simulink model "feedback_control_basic"  (R2017a)
settings: Solver=VariableStepAuto  StartTime=0.0  StopTime=10.0  RelTol=1e-3
libraries: cstblocks x5
settings Model: Creator=Roman  LastModifiedBy=Roman

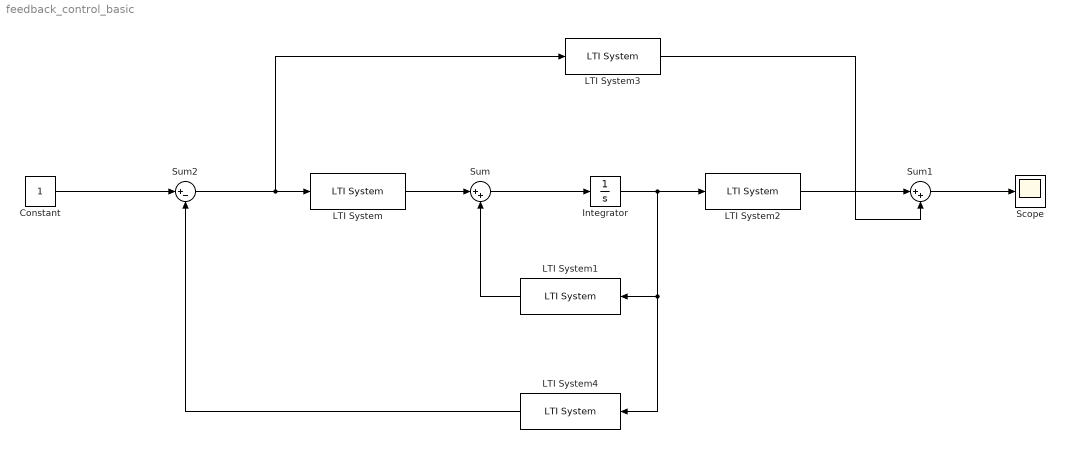
== system feedback_control_basic ==
  Constant : Constant
  Integrator : Integrator
  LTI System : cstblocks/LTI System  sys=B  IC=[]
  LTI System1 : cstblocks/LTI System  sys=A  IC=[]
  LTI System2 : cstblocks/LTI System  sys=C  IC=[]
  LTI System3 : cstblocks/LTI System  sys=D  IC=[]
  LTI System4 : cstblocks/LTI System  sys=K  IC=[]
  Scope : Scope
  Sum : Sum  Inputs=|++
  Sum1 : Sum  Inputs=|++
  Sum2 : Sum  Inputs=|+-
  wires:
  Integrator/1 -> LTI System4/1, LTI System1/1, LTI System2/1
  LTI System1/1 -> Sum/2
  LTI System/1 -> Sum/1
  Sum/1 -> Integrator/1
  LTI System2/1 -> Sum1/1
  LTI System3/1 -> Sum1/2
  Sum1/1 -> Scope/1
  LTI System4/1 -> Sum2/2
  Sum2/1 -> LTI System3/1, LTI System/1
  Constant/1 -> Sum2/1
